simulink model "sweep_testbench"  (R2021b)
settings: Solver=FixedStepDiscrete  StartTime=0.0  StopTime=swpctrl.trantime  FixedStep=1/Fs  RelTol=1e-3  EnableMultiTasking=on
undefined symbols (not defined in the file): Fs, input_dc, sinamp, sinfreq, swpctrl
libraries: dspsrcs4 x1
settings Model: Creator=amyles  LastModifiedBy=91573
settings SolverCC: AlgebraicLoopSolver=TrustRegion
settings DataIOCC: SaveFormat=Array  SignalLoggingSaveFormat=ModelDataLogs  ReturnWorkspaceOutputs=off
settings OptimizationCC: ExpressionDepthLimit=2147483647  LifeSpan=inf
settings DebuggingCC: UnderspecifiedInitializationDetection=Classic  MergeDetectMultiDrivingBlocksExec=none  SolverPrmCheckMsg=warning  FcnCallInpInsideContextMsg=warning  StateNameClashWarn=warning  SFUnexpectedBacktrackingDiag=warning  SFNoUnconditionalDefaultTransitionDiag=warning  SFExecutionAtInitializationDiag=none  SFMachineParentedDataDiag=warning  ArithmeticOperatorsInVariantConditions=warning
settings HardwareCC: ProdBitPerPointer=32  ProdBitPerSizeT=32  ProdBitPerPtrDiffT=32  ProdLargestAtomicFloat=None  ProdIntDivRoundTo=Undefined  ProdEndianess=Unspecified  ProdWordSize=32  ProdHWDeviceType=32-bit Generic
settings ModelReferenceCC: ModelReferenceNumInstancesAllowed=Single  PropagateSignalLabelsOutOfModel=off
settings SFSimCC: SimUseLocalCustomCode=off  CustomCodeUndefinedFunction=UseInterfaceOnly
settings RTWCC: RTWUseLocalCustomCode=off
settings CodeAppCC: StateflowObjectComments=on
settings GRTTargetCC: TargetLangStandard=C89/C90 (ANSI)  CombineOutputUpdateFcns=off  GRTInterface=on
settings ConfigComp: CovMetricSettings=dw  CovSaveCumulativeToWorkspaceVar=on  CovSaveSingleToWorkspaceVar=on  CovExternalEMLEnable=off

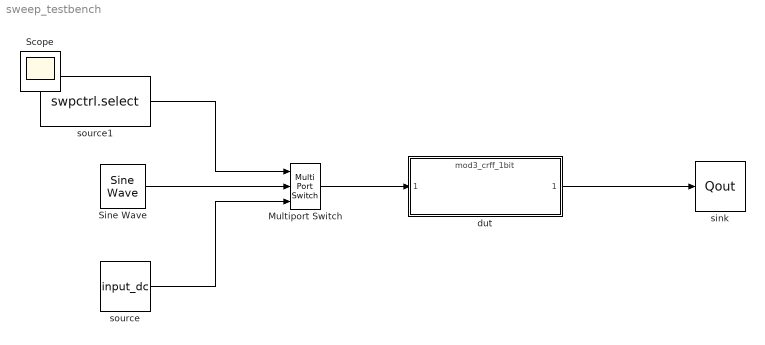
== system sweep_testbench ==
  Multiport Switch : MultiPortSwitch  Inputs=2
  Sine Wave : dspsrcs4/Sine Wave  Amplitude=sinamp  Frequency=sinfreq  Phase=0  SampleMode=Discrete  OutComplex=Real  CompMethod=Trigonometric fcn  TableSize=Speed  SampleTime=1/Fs  SamplesPerFrame=1  ResetState=Restart at time zero  OutputFrames=on  dataType=double  wordLen=16  udDataType=sfix(16)  fracBitsMode=Best precision  numFracBits=15  OutDataTypeStr=double  LastOutDataTypeStr=double
  dut : ModelReference  ModelNameDialog=mod3_crff_1bit.mdl  SimulationMode=Normal  ModelReferenceVersion=1.97
  sink : ToWorkspace  VariableName=Qout  SampleTime=-1
      settings: MaxDataPoints=50000000
  source : Constant  Value=input_dc  SampleTime=1/Fs
  source1 : Constant  Value=swpctrl.select  SampleTime=1/Fs
  Scope : Scope
  wires:
  Multiport Switch/1 -> dut/1
  Sine Wave/1 -> Multiport Switch/2
  source/1 -> Multiport Switch/3
  source1/1 -> Multiport Switch/1
  dut/1 -> sink/1
